simulink subsystem "Rotor_Gyroscopic_Loads"  (R2021b)
settings: Solver=VariableStepAuto  StartTime=0.0  StopTime=10.0  RelTol=1e-3
settings Model: DefaultTestHarness=Rotor_Gyroscopic_Loads_ValidationV1  Creator=PhilippSchildt  LastModifiedBy=PhilippSchildt
settings SolverCC: AlgebraicLoopSolver=TrustRegion
settings DebuggingCC: SFMachineParentedDataDiag=warning

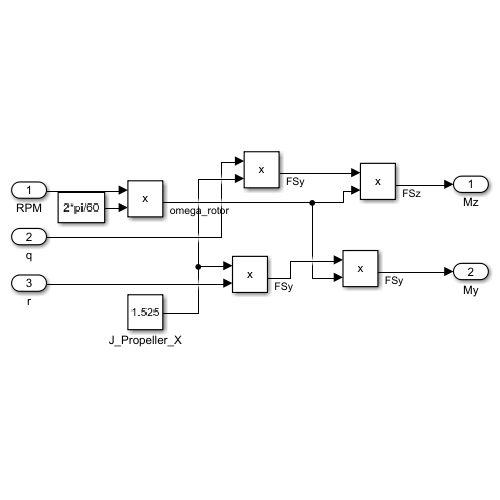
[thumbnail: Simulink's stored preview of the top-level diagram]
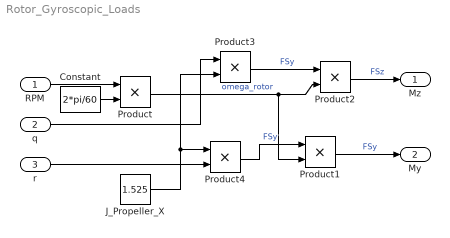
== system Rotor_Gyroscopic_Loads ==
  RPM : Inport
  q : Inport  Port=2
  r : Inport  Port=3
  Constant : Constant  Value=2*pi/60
  J_Propeller_X : Constant  Value=1.525
  Product{,1..4} (5 alike) : Product
  Mz : Outport
  My : Outport  Port=2
  wires:
  RPM/1 -> Product/1
  Constant/1 -> Product/2
  Product2/1 -> Mz/1  "FSz"
  Product1/1 -> My/1  "FSy"
  Product4/1 -> Product1/1  "FSy"
  Product3/1 -> Product2/1  "FSy"
  Product/1 -> Product2/2, Product1/2  "omega_rotor"
  r/1 -> Product4/2
  J_Propeller_X/1 -> Product3/2, Product4/1
  q/1 -> Product3/1
